simulink model "simTest"  (R2015a)
settings: Solver=ode45  StartTime=0.0  StopTime=10.0  RelTol=1e-3
libraries: simulink x1
settings Model: Creator=JoshuaLevy  LastModifiedBy=JoshuaLevy

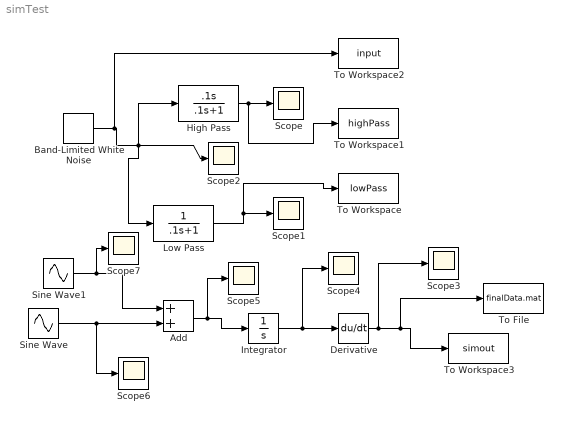
== system simTest ==
  Add : Sum
  Band-Limited White Noise : simulink/Sources/Band-Limited White Noise  Cov=[0.1]  Ts=0.1  seed=[23341]
  Derivative : Derivative
  High Pass : TransferFcn  Numerator=[.1 0]  Denominator=[.1 1]
  Integrator : Integrator  LimitOutput=on
  Low Pass : TransferFcn  Denominator=[.1 1]
  Scope{,1..7} (8 alike) : Scope
      Scope2 settings: SaveName=ScopeData2
      Scope3 settings: SaveName=ScopeData3
      Scope4 settings: SaveName=ScopeData4
      Scope5 settings: SaveName=ScopeData5
      Scope6 settings: SaveName=ScopeData6
      Scope7 settings: SaveName=ScopeData7
  Sine Wave : Sin  Amplitude=3  Frequency=2  Phase=1  SampleTime=0
  Sine Wave1 : Sin  Amplitude=2  Frequency=5  Phase=4.5685  SampleTime=0
  To File : ToFile  Filename=finalData.mat  SaveFormat=Timeseries
  To Workspace : ToWorkspace  VariableName=lowPass  SaveFormat=Timeseries  SampleTime=-1
  To Workspace1 : ToWorkspace  VariableName=highPass  SaveFormat=Timeseries  SampleTime=-1
  To Workspace2 : ToWorkspace  VariableName=input  SaveFormat=Timeseries  SampleTime=-1
  To Workspace3 : ToWorkspace  VariableName=simout  SaveFormat=Timeseries  SampleTime=-1
  wires:
  Band-Limited White Noise/1 -> To Workspace2/1, Low Pass/1, Scope2/1, High Pass/1
  High Pass/1 -> To Workspace1/1, Scope/1
  Low Pass/1 -> To Workspace/1, Scope1/1
  Sine Wave1/1 -> Scope7/1, Add/1
  Sine Wave/1 -> Scope6/1, Add/2
  Add/1 -> Scope5/1, Integrator/1
  Integrator/1 -> Scope4/1, Derivative/1
  Derivative/1 -> Scope3/1, To File/1, To Workspace3/1
